simulink model "mrefrobotarm_previous_y_previous_u_previous_ref_cex_2"  (R2018b)
settings: Solver=FixedStepAuto  StartTime=0.0  StopTime=20  RelTol=1e-3  AbsTol=1e-6
undefined symbols (not defined in the file or in its folder): cc, options
libraries: neural x462, simulink x2
(part 8 of 18)

== system mrefrobotarm_previous_y_previous_u_previous_ref_cex_2/cex_m1/Layer 3/Delays 1 ==
  "p{3}" : Inport  PortDimensions=30
      mask Display: e = 0.06;c1 = [120 230 180]/255;c2 = ([120 230 180]+0)/(256+128);c3 = ([120 230 180]+128)/(256+128);patch([0 1 1 0],[0 0 1 1],c1);patch([0 1 1 1-e 1-e 0+e],[0 0 1 1-e 0+e 0+e],c2);patch([0 0 1 1-e 0+e 0+e],[0 1 1 1-e 1-e 0+e],c3);plot([0 1 1 0 0],[0 0 1 1 0]);
  mux : Mux  Inputs=1
      mask Display: e = 0.06;c1 = [120 150 230]/255;c2 = ([120 150 230]+0)/383;c3 = ([120 150 230]+128)/383;patch([0 1 1 0],[0 0 1 1],c1);patch([0 1 1 1-e 1-e 0+e],[0 0 1 1-e 0+e 0+e],c2);patch([0 0 1 1-e 0+e 0+e],[0 1 1 1-e 1-e 0+e],c3);plot([0 1 1 0 0],[0 0 1 1 0]);disp('Mux')
  "pd{3,2}" : Outport
      mask Display: e = 0.06;c1 = [120 230 180]/255;c2 = ([120 230 180]+0)/(256+128);c3 = ([120 230 180]+128)/(256+128);patch([0 1 1 0],[0 0 1 1],c1);patch([0 1 1 1-e 1-e 0+e],[0 0 1 1-e 0+e 0+e],c2);patch([0 0 1 1-e 0+e 0+e],[0 1 1 1-e 1-e 0+e],c3);plot([0 1 1 0 0],[0 0 1 1 0]);
  wires:
  "p{3}"/1 -> mux/1
  mux/1 -> "pd{3,2}"/1

== system mrefrobotarm_previous_y_previous_u_previous_ref_cex_2/cex_m1/Layer 3/LW{3,2} ==
  "ad{3,2}" : Inport  PortDimensions=30
      mask Display: e = 0.06;c1 = [120 230 180]/255;c2 = ([120 230 180]+0)/(256+128);c3 = ([120 230 180]+128)/(256+128);patch([0 1 1 0],[0 0 1 1],c1);patch([0 1 1 1-e 1-e 0+e],[0 0 1 1-e 0+e 0+e],c2);patch([0 0 1 1-e 0+e 0+e],[0 1 1 1-e 1-e 0+e],c3);plot([0 1 1 0 0],[0 0 1 1 0]);
  "IW{3,2}(1,:)'" : Constant  Value=[0.273559337497494947655241048778407275676727294921875;-0.7756545835412576028744524592184461653232574462890625;-0.2367085924296140897471474318081163801252841949462890625;-0.07780558994367196834485156387017923407256603240966796875;0.62547021966759819289194410885102115571498870849609375;-0.042949116212649039725501864950274466536939144134521484375;-0.0115378064817653024076715695400707772932946681976318359375;-0.1916034773301610594220534267151379026472568511962890625;0.07545572263788587197286261698536691255867481231689453125;-0.342221555072600935876181438288767822086811065673828125;0.05574493159312048085052282431206549517810344696044921875;-0.118390555813133235840695078877615742385387420654296875;0.405364924953283967123951470057363621890544891357421875;-0.62424190657044953400856002190266735851764678955078125;0.267676026784579856876433723300579003989696502685546875;-0.53578877848254624627344355758395977318286895751953125;-0.393016319594194307729395632122759707272052764892578125;0.204836160849805881678520336208748631179332733154296875;0.1641507664097359986410396004430367611348628997802734375;0.34723625620254361390237818341120146214962005615234375;0.00875153796303594112837576091123992227949202060699462890625;-0.035480681395222139762335444856944377534091472625732421875;0.021397552117908107127686179183001513592898845672607421875;-0.300775979439210860988396234461106359958648681640625;-0.277260526293208686698932297076680697500705718994140625;-0.09496793333009435900127215290922322310507297515869140625;0.01226152538563072928734509758896820130757987499237060546875;0.051278382491689360189734969708297285251319408416748046875;0.86445975923971551946323188531096093356609344482421875;-0.36925297458121264515540360662271268665790557861328125]
      mask Display: e = 0.06;c1 = [120 150 230]/255;c2 = ([120 150 230]+0)/383;c3 = ([120 150 230]+128)/383;patch([0 1 1 0],[0 0 1 1],c1);patch([0 1 1 1-e 1-e 0+e],[0 0 1 1-e 0+e 0+e],c2);patch([0 0 1 1-e 0+e 0+e],[0 1 1 1-e 1-e 0+e],c3);plot([0 1 1 0 0],[0 0 1 1 0]);disp('weights');
  Mux : Mux  Inputs=1
      mask Display: e = 0.06;c1 = [120 150 230]/255;c2 = ([120 150 230]+0)/383;c3 = ([120 150 230]+128)/383;patch([0 1 1 0],[0 0 1 1],c1);patch([0 1 1 1-e 1-e 0+e],[0 0 1 1-e 0+e 0+e],c2);patch([0 0 1 1-e 0+e 0+e],[0 1 1 1-e 1-e 0+e],c3);plot([0 1 1 0 0],[0 0 1 1 0]);disp('Mux');
  dotprod1 : neural/Weight Functions/dotprod
  "lz{3,2}" : Outport
      mask Display: e = 0.06;c1 = [120 230 180]/255;c2 = ([120 230 180]+0)/(256+128);c3 = ([120 230 180]+128)/(256+128);patch([0 1 1 0],[0 0 1 1],c1);patch([0 1 1 1-e 1-e 0+e],[0 0 1 1-e 0+e 0+e],c2);patch([0 0 1 1-e 0+e 0+e],[0 1 1 1-e 1-e 0+e],c3);plot([0 1 1 0 0],[0 0 1 1 0]);
  wires:
  "IW{3,2}(1,:)'"/1 -> dotprod1/1
  "ad{3,2}"/1 -> dotprod1/2
  dotprod1/1 -> Mux/1
  Mux/1 -> "lz{3,2}"/1

== system mrefrobotarm_previous_y_previous_u_previous_ref_cex_2/cex_m1_old/Layer 1/Delays 1 ==
  "p{1}" : Inport  PortDimensions=10
      mask Display: e = 0.06;c1 = [120 230 180]/255;c2 = ([120 230 180]+0)/(256+128);c3 = ([120 230 180]+128)/(256+128);patch([0 1 1 0],[0 0 1 1],c1);patch([0 1 1 1-e 1-e 0+e],[0 0 1 1-e 0+e 0+e],c2);patch([0 0 1 1-e 0+e 0+e],[0 1 1 1-e 1-e 0+e],c3);plot([0 1 1 0 0],[0 0 1 1 0]);
  mux : Mux  Inputs=1
      mask Display: e = 0.06;c1 = [120 150 230]/255;c2 = ([120 150 230]+0)/383;c3 = ([120 150 230]+128)/383;patch([0 1 1 0],[0 0 1 1],c1);patch([0 1 1 1-e 1-e 0+e],[0 0 1 1-e 0+e 0+e],c2);patch([0 0 1 1-e 0+e 0+e],[0 1 1 1-e 1-e 0+e],c3);plot([0 1 1 0 0],[0 0 1 1 0]);disp('Mux')
  "pd{1,1}" : Outport
      mask Display: e = 0.06;c1 = [120 230 180]/255;c2 = ([120 230 180]+0)/(256+128);c3 = ([120 230 180]+128)/(256+128);patch([0 1 1 0],[0 0 1 1],c1);patch([0 1 1 1-e 1-e 0+e],[0 0 1 1-e 0+e 0+e],c2);patch([0 0 1 1-e 0+e 0+e],[0 1 1 1-e 1-e 0+e],c3);plot([0 1 1 0 0],[0 0 1 1 0]);
  wires:
  "p{1}"/1 -> mux/1
  mux/1 -> "pd{1,1}"/1

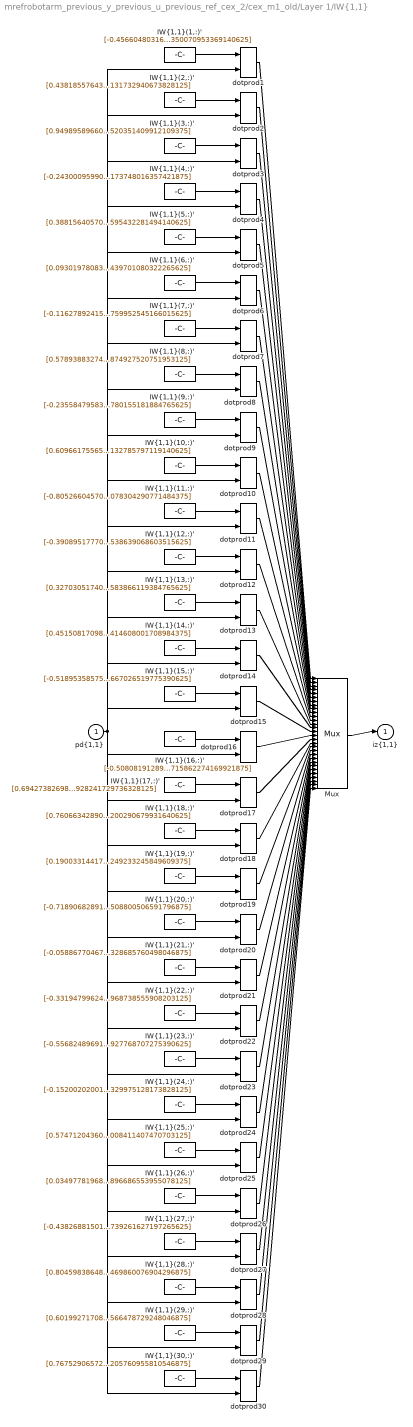
== system mrefrobotarm_previous_y_previous_u_previous_ref_cex_2/cex_m1_old/Layer 1/IW{1,1} ==
  "pd{1,1}" : Inport  PortDimensions=10
      mask Display: e = 0.06;c1 = [120 230 180]/255;c2 = ([120 230 180]+0)/(256+128);c3 = ([120 230 180]+128)/(256+128);patch([0 1 1 0],[0 0 1 1],c1);patch([0 1 1 1-e 1-e 0+e],[0 0 1 1-e 0+e 0+e],c2);patch([0 0 1 1-e 0+e 0+e],[0 1 1 1-e 1-e 0+e],c3);plot([0 1 1 0 0],[0 0 1 1 0]);
  "IW{1,1}(1,:)'" : Constant  Value=[-0.456604803168614292729898807010613381862640380859375;-0.337127164338302864887708665264653973281383514404296875;-0.09380605620231612096215911833496647886931896209716796875;0.4813255060015799724482121746405027806758880615234375;-0.51828644978876658999666915406123735010623931884765625;-0.360214664462510547604523480913485400378704071044921875;-0.1613924539391769774621110400403267703950405120849609375;-0.45837538185699278070472928447998128831386566162109375;0.98037037066747012570289143695845268666744232177734375;0.369741124667328835418089738595881499350070953369140625]
      mask Display: e = 0.06;c1 = [120 150 230]/255;c2 = ([120 150 230]+0)/383;c3 = ([120 150 230]+128)/383;patch([0 1 1 0],[0 0 1 1],c1);patch([0 1 1 1-e 1-e 0+e],[0 0 1 1-e 0+e 0+e],c2);patch([0 0 1 1-e 0+e 0+e],[0 1 1 1-e 1-e 0+e],c3);plot([0 1 1 0 0],[0 0 1 1 0]);disp('Weights');
  "IW{1,1}(10,:)'" : Constant  Value=[0.60966175565233104993723145526018925011157989501953125;-0.78590103009985778914625598190468735992908477783203125;0.67529278324963026847171931876800954341888427734375;-0.538121168742959010700133148930035531520843505859375;0.6927400264329157675291526174987666308879852294921875;0.340750317165999572210921542136929929256439208984375;0.40556995495471770407647227330016903579235076904296875;-0.0484033308948597085219489599694497883319854736328125;-0.164300434052266519646678943900042213499546051025390625;-0.58676709523571946025555234882631339132785797119140625]
      mask Display: e = 0.06;c1 = [120 150 230]/255;c2 = ([120 150 230]+0)/383;c3 = ([120 150 230]+128)/383;patch([0 1 1 0],[0 0 1 1],c1);patch([0 1 1 1-e 1-e 0+e],[0 0 1 1-e 0+e 0+e],c2);patch([0 0 1 1-e 0+e 0+e],[0 1 1 1-e 1-e 0+e],c3);plot([0 1 1 0 0],[0 0 1 1 0]);disp('Weights');
  "IW{1,1}(11,:)'" : Constant  Value=[-0.8052660457061115995003319767420180141925811767578125;-0.390578940383738970609783791587688028812408447265625;-0.307426974497562233157310629394487477838993072509765625;0.18849807820618769138576453769928775727748870849609375;-0.39029554181874825946607643345487304031848907470703125;0.50189857658144487739804162629297934472560882568359375;-1.3944440472362054084243254692410118877887725830078125;0.052818878114326554829016657777174259535968303680419921875;0.52703996195776647848418861030950210988521575927734375;0.64912684710533896659256924976943992078304290771484375]
      mask Display: e = 0.06;c1 = [120 150 230]/255;c2 = ([120 150 230]+0)/383;c3 = ([120 150 230]+128)/383;patch([0 1 1 0],[0 0 1 1],c1);patch([0 1 1 1-e 1-e 0+e],[0 0 1 1-e 0+e 0+e],c2);patch([0 0 1 1-e 0+e 0+e],[0 1 1 1-e 1-e 0+e],c3);plot([0 1 1 0 0],[0 0 1 1 0]);disp('Weights');
  "IW{1,1}(12,:)'" : Constant  Value=[-0.39089517770435111554405693823355250060558319091796875;0.87652548903037030836316034765332005918025970458984375;-0.86066296477683745802522707890602760016918182373046875;0.2435082234393515232540039505693130195140838623046875;-0.01260654893496855090406771893185577937401831150054931640625;0.58088923822424043397205650762771256268024444580078125;0.79790414878794369002434905269183218479156494140625;-0.321088353238704937719916188143542967736721038818359375;0.46829250187147308803758960493723861873149871826171875;0.105276077235084086769489886137307621538639068603515625]
      mask Display: e = 0.06;c1 = [120 150 230]/255;c2 = ([120 150 230]+0)/383;c3 = ([120 150 230]+128)/383;patch([0 1 1 0],[0 0 1 1],c1);patch([0 1 1 1-e 1-e 0+e],[0 0 1 1-e 0+e 0+e],c2);patch([0 0 1 1-e 0+e 0+e],[0 1 1 1-e 1-e 0+e],c3);plot([0 1 1 0 0],[0 0 1 1 0]);disp('Weights');
  "IW{1,1}(13,:)'" : Constant  Value=[0.327030517403528120379263555150828324258327484130859375;-0.85196641992506927376638259374885819852352142333984375;-0.3458136539724006031093495039385743439197540283203125;0.56880574832738928225950303385616280138492584228515625;0.060222487967785363893735706142251729033887386322021484375;0.0444849469077064352262596003129146993160247802734375;-0.6806078651776008570095655159093439579010009765625;0.443959968651114367244048253269284032285213470458984375;-0.23601846855789110346535153439617715775966644287109375;0.60569342459776598364129540641442872583866119384765625]
      mask Display: e = 0.06;c1 = [120 150 230]/255;c2 = ([120 150 230]+0)/383;c3 = ([120 150 230]+128)/383;patch([0 1 1 0],[0 0 1 1],c1);patch([0 1 1 1-e 1-e 0+e],[0 0 1 1-e 0+e 0+e],c2);patch([0 0 1 1-e 0+e 0+e],[0 1 1 1-e 1-e 0+e],c3);plot([0 1 1 0 0],[0 0 1 1 0]);disp('Weights');
  "IW{1,1}(14,:)'" : Constant  Value=[0.4515081709834014578319738575373776257038116455078125;-0.8989078222605810797318781624198891222476959228515625;0.454253767808243280601487867897958494722843170166015625;-0.197872388974969226627109719629515893757343292236328125;-0.284539642220156763219307549661607481539249420166015625;0.8759306435735558782340604011551477015018463134765625;-0.1785360111457083842623205782729201018810272216796875;-0.2001588807255618995828427841843222267925739288330078125;0.53520676898232066864835587693960405886173248291015625;0.94559736423401774541019904063432477414608001708984375]
      mask Display: e = 0.06;c1 = [120 150 230]/255;c2 = ([120 150 230]+0)/383;c3 = ([120 150 230]+128)/383;patch([0 1 1 0],[0 0 1 1],c1);patch([0 1 1 1-e 1-e 0+e],[0 0 1 1-e 0+e 0+e],c2);patch([0 0 1 1-e 0+e 0+e],[0 1 1 1-e 1-e 0+e],c3);plot([0 1 1 0 0],[0 0 1 1 0]);disp('Weights');
  "IW{1,1}(15,:)'" : Constant  Value=[-0.518953585756852131538607864058576524257659912109375;-0.8287693770535684567590806182124651968479156494140625;0.61069653280025570918354560490115545690059661865234375;0.455111773439323352707930325777851976454257965087890625;0.61500607296115672451009004362276755273342132568359375;-0.36577833850321705977393094144645147025585174560546875;0.1471285663392648823677433256307267583906650543212890625;-0.5784088886907132742720705209649167954921722412109375;0.07806634820889439552171751302012125961482524871826171875;0.69003575602860645066272127223783172667026519775390625]
      mask Display: e = 0.06;c1 = [120 150 230]/255;c2 = ([120 150 230]+0)/383;c3 = ([120 150 230]+128)/383;patch([0 1 1 0],[0 0 1 1],c1);patch([0 1 1 1-e 1-e 0+e],[0 0 1 1-e 0+e 0+e],c2);patch([0 0 1 1-e 0+e 0+e],[0 1 1 1-e 1-e 0+e],c3);plot([0 1 1 0 0],[0 0 1 1 0]);disp('Weights');
  "IW{1,1}(16,:)'" : Constant  Value=[-0.5080819128972311471414968764293007552623748779296875;0.064120829622686448256985158877796493470668792724609375;-0.1899203040905295403195651715577696450054645538330078125;0.028825660348881392003317358785352553240954875946044921875;0.8950447302793678172605496001779101788997650146484375;-0.6350696078018034373968703221180476248264312744140625;0.69836883039490371682944669373682700097560882568359375;-0.2994246938013576109227642518817447125911712646484375;0.56725449704477826085025071733980439603328704833984375;-0.37050563293872595949096648837439715862274169921875]
      mask Display: e = 0.06;c1 = [120 150 230]/255;c2 = ([120 150 230]+0)/383;c3 = ([120 150 230]+128)/383;patch([0 1 1 0],[0 0 1 1],c1);patch([0 1 1 1-e 1-e 0+e],[0 0 1 1-e 0+e 0+e],c2);patch([0 0 1 1-e 0+e 0+e],[0 1 1 1-e 1-e 0+e],c3);plot([0 1 1 0 0],[0 0 1 1 0]);disp('Weights');
  "IW{1,1}(17,:)'" : Constant  Value=[0.69427382698219963774732832462177611887454986572265625;-0.488497940847307077216754578330437652766704559326171875;0.76921833962025198960787975011044181883335113525390625;-0.91091754430127747088619116766494698822498321533203125;-0.1745040246724469945593938291494851000607013702392578125;0.0066101774826527737172199294946040026843547821044921875;0.453900939435363082186114525029552169144153594970703125;0.07387565171452577239552539367650751955807209014892578125;0.69920054733834613447385208928608335554599761962890625;-0.1244791951685582376274652460779179818928241729736328125]
      mask Display: e = 0.06;c1 = [120 150 230]/255;c2 = ([120 150 230]+0)/383;c3 = ([120 150 230]+128)/383;patch([0 1 1 0],[0 0 1 1],c1);patch([0 1 1 1-e 1-e 0+e],[0 0 1 1-e 0+e 0+e],c2);patch([0 0 1 1-e 0+e 0+e],[0 1 1 1-e 1-e 0+e],c3);plot([0 1 1 0 0],[0 0 1 1 0]);disp('Weights');
  "IW{1,1}(18,:)'" : Constant  Value=[0.76066342890209115434885234208195470273494720458984375;0.51801825655466082753974887964432127773761749267578125;0.91420683388085322018667966403882019221782684326171875;-0.49680504344115739012721633116598241031169891357421875;0.926993167798115802469283153186552226543426513671875;0.38135095924055273375330443741404451429843902587890625;0.774530566058326375156184440129436552524566650390625;-0.533047430909843189539287777733989059925079345703125;-0.0174997496667618490651108231759280897676944732666015625;0.355609156460071462735328395865508355200290679931640625]
      mask Display: e = 0.06;c1 = [120 150 230]/255;c2 = ([120 150 230]+0)/383;c3 = ([120 150 230]+128)/383;patch([0 1 1 0],[0 0 1 1],c1);patch([0 1 1 1-e 1-e 0+e],[0 0 1 1-e 0+e 0+e],c2);patch([0 0 1 1-e 0+e 0+e],[0 1 1 1-e 1-e 0+e],c3);plot([0 1 1 0 0],[0 0 1 1 0]);disp('Weights');
  "IW{1,1}(19,:)'" : Constant  Value=[0.1900331441796630771445819618747918866574764251708984375;0.53025746047892752255137338579515926539897918701171875;-0.395669897903047240728113820296130143105983734130859375;-0.6907448236475797198608006510767154395580291748046875;0.36487531515756810307493651635013520717620849609375;-0.84679918588567992809856832536752335727214813232421875;0.292288624186119172509989994068746455013751983642578125;0.1586375850129098097340829554013907909393310546875;0.041807865616759622151565878311885171569883823394775390625;0.95747807301410892133475272203213535249233245849609375]
      mask Display: e = 0.06;c1 = [120 150 230]/255;c2 = ([120 150 230]+0)/383;c3 = ([120 150 230]+128)/383;patch([0 1 1 0],[0 0 1 1],c1);patch([0 1 1 1-e 1-e 0+e],[0 0 1 1-e 0+e 0+e],c2);patch([0 0 1 1-e 0+e 0+e],[0 1 1 1-e 1-e 0+e],c3);plot([0 1 1 0 0],[0 0 1 1 0]);disp('Weights');
  "IW{1,1}(2,:)'" : Constant  Value=[0.438185576430030920835889673981000669300556182861328125;0.63169008794116454641454083684948273003101348876953125;-0.690212126796364344727408024482429027557373046875;0.126418981169538924280715264103491790592670440673828125;-0.78081879756354766186632332392036914825439453125;0.036441711512395225103233542540692724287509918212890625;0.80831443252255363862701642574393190443515777587890625;-0.5695381261843135423106332382303662598133087158203125;0.372937259042779134521339301500120200216770172119140625;0.76200855637333220204965300581534393131732940673828125]
      mask Display: e = 0.06;c1 = [120 150 230]/255;c2 = ([120 150 230]+0)/383;c3 = ([120 150 230]+128)/383;patch([0 1 1 0],[0 0 1 1],c1);patch([0 1 1 1-e 1-e 0+e],[0 0 1 1-e 0+e 0+e],c2);patch([0 0 1 1-e 0+e 0+e],[0 1 1 1-e 1-e 0+e],c3);plot([0 1 1 0 0],[0 0 1 1 0]);disp('Weights');
  "IW{1,1}(20,:)'" : Constant  Value=[-0.71890682891750745664438682069885544478893280029296875;0.323748238412146893683285497900214977562427520751953125;-0.4350383245811233479116708622314035892486572265625;-0.098115153846664859838000438685412518680095672607421875;0.332374149245302785704581083336961455643177032470703125;0.665347500692802018562588273198343813419342041015625;-0.996297270814632707214286710950545966625213623046875;0.22478310077883134621146155041060410439968109130859375;0.07675674847099771269665069439724902622401714324951171875;-0.39635430828158735305777327084797434508800506591796875]
      mask Display: e = 0.06;c1 = [120 150 230]/255;c2 = ([120 150 230]+0)/383;c3 = ([120 150 230]+128)/383;patch([0 1 1 0],[0 0 1 1],c1);patch([0 1 1 1-e 1-e 0+e],[0 0 1 1-e 0+e 0+e],c2);patch([0 0 1 1-e 0+e 0+e],[0 1 1 1-e 1-e 0+e],c3);plot([0 1 1 0 0],[0 0 1 1 0]);disp('Weights');
  "IW{1,1}(21,:)'" : Constant  Value=[-0.058867704679459571803779027732161921449005603790283203125;0.318806140277555438711232227433356456458568572998046875;0.5514498503440876664427605646778829395771026611328125;-0.843025654861124795758087202557362616062164306640625;0.42766102343846423838868986422312445938587188720703125;-0.73504404909710008286793936349567957222461700439453125;-0.76913120987454008936623495173989795148372650146484375;0.0070151290944123097237383746005434659309685230255126953125;0.79142247809240073852521391017944552004337310791015625;0.283648015671342956789402478534611873328685760498046875]
      mask Display: e = 0.06;c1 = [120 150 230]/255;c2 = ([120 150 230]+0)/383;c3 = ([120 150 230]+128)/383;patch([0 1 1 0],[0 0 1 1],c1);patch([0 1 1 1-e 1-e 0+e],[0 0 1 1-e 0+e 0+e],c2);patch([0 0 1 1-e 0+e 0+e],[0 1 1 1-e 1-e 0+e],c3);plot([0 1 1 0 0],[0 0 1 1 0]);disp('Weights');
  "IW{1,1}(22,:)'" : Constant  Value=[-0.331947996244390031161941578830010257661342620849609375;-0.2268747378868123387718469530227594077587127685546875;0.61424614718336278951227313882554881274700164794921875;-0.57641523587598830768996549522853456437587738037109375;-0.6983402399747113964423306242679245769977569580078125;0.73226198126729824533498458549729548394680023193359375;0.6098680765245083623682376128272153437137603759765625;-0.81514112188509824097337741477531380951404571533203125;0.5435968206353025689026026157080195844173431396484375;0.383290174564916708010997581368428654968738555908203125]
      mask Display: e = 0.06;c1 = [120 150 230]/255;c2 = ([120 150 230]+0)/383;c3 = ([120 150 230]+128)/383;patch([0 1 1 0],[0 0 1 1],c1);patch([0 1 1 1-e 1-e 0+e],[0 0 1 1-e 0+e 0+e],c2);patch([0 0 1 1-e 0+e 0+e],[0 1 1 1-e 1-e 0+e],c3);plot([0 1 1 0 0],[0 0 1 1 0]);disp('Weights');
  "IW{1,1}(23,:)'" : Constant  Value=[-0.55682489691597714109860817188746295869350433349609375;0.3971753371402726440209107749979011714458465576171875;-0.94266284346768802748783855349756777286529541015625;0.2233454508858634113277474853020976297557353973388671875;-0.78108602978100460934030024873209185898303985595703125;-0.355621419148077710925548444720334373414516448974609375;1.04371286491103543170311240828596055507659912109375;-0.575221360774758050382615692797116935253143310546875;-0.040419337166701672925395172342177829705178737640380859375;0.60627576039757935522089837832027114927768707275390625]
      mask Display: e = 0.06;c1 = [120 150 230]/255;c2 = ([120 150 230]+0)/383;c3 = ([120 150 230]+128)/383;patch([0 1 1 0],[0 0 1 1],c1);patch([0 1 1 1-e 1-e 0+e],[0 0 1 1-e 0+e 0+e],c2);patch([0 0 1 1-e 0+e 0+e],[0 1 1 1-e 1-e 0+e],c3);plot([0 1 1 0 0],[0 0 1 1 0]);disp('Weights');
  "IW{1,1}(24,:)'" : Constant  Value=[-0.152002020012920124880650973864248953759670257568359375;0.267355262853008091017414926682249642908573150634765625;0.3681014583243105153798069295589812099933624267578125;0.60380396349835752101142816172796301543712615966796875;-0.2240663683106254300270165913389064371585845947265625;-0.2118074012804891104178039995531435124576091766357421875;0.61766038108176901655355095499544404447078704833984375;-0.10347664558279710822485952803617692552506923675537109375;1.0088377721471577519452011983958072960376739501953125;-0.296533638802529697642285100300796329975128173828125]
      mask Display: e = 0.06;c1 = [120 150 230]/255;c2 = ([120 150 230]+0)/383;c3 = ([120 150 230]+128)/383;patch([0 1 1 0],[0 0 1 1],c1);patch([0 1 1 1-e 1-e 0+e],[0 0 1 1-e 0+e 0+e],c2);patch([0 0 1 1-e 0+e 0+e],[0 1 1 1-e 1-e 0+e],c3);plot([0 1 1 0 0],[0 0 1 1 0]);disp('Weights');
  "IW{1,1}(25,:)'" : Constant  Value=[0.5747120436081643024550658083171583712100982666015625;-1.0586365897313012585101432705414481461048126220703125;0.09387458902065796972902234074354055337607860565185546875;-0.052016654662084292615187308683744049631059169769287109375;-0.4780536664053312012612195758265443146228790283203125;0.9806526512700610709316606516949832439422607421875;-0.1030533823984588204236700903493328951299190521240234375;-0.16531964088011064095695701325894333422183990478515625;0.32575705366995766354420993593521416187286376953125;-0.8915608655361009216022694090497680008411407470703125]
      mask Display: e = 0.06;c1 = [120 150 230]/255;c2 = ([120 150 230]+0)/383;c3 = ([120 150 230]+128)/383;patch([0 1 1 0],[0 0 1 1],c1);patch([0 1 1 1-e 1-e 0+e],[0 0 1 1-e 0+e 0+e],c2);patch([0 0 1 1-e 0+e 0+e],[0 1 1 1-e 1-e 0+e],c3);plot([0 1 1 0 0],[0 0 1 1 0]);disp('Weights');
  "IW{1,1}(26,:)'" : Constant  Value=[0.0349778196856112277846051483720657415688037872314453125;1.0546893984497180962733864362235181033611297607421875;0.5113372359302978953365936831687577068805694580078125;-0.20958359966499229276593041504384018480777740478515625;-0.45906996765058216691812731369282118976116180419921875;-0.350427826420348365044077354468754492700099945068359375;0.91643043413432445642996526657952927052974700927734375;-0.6214855448244855917749873697175644338130950927734375;-0.52581356029745618396731288157752715051174163818359375;-0.06278736980947492718474478579082642681896686553955078125]
      mask Display: e = 0.06;c1 = [120 150 230]/255;c2 = ([120 150 230]+0)/383;c3 = ([120 150 230]+128)/383;patch([0 1 1 0],[0 0 1 1],c1);patch([0 1 1 1-e 1-e 0+e],[0 0 1 1-e 0+e 0+e],c2);patch([0 0 1 1-e 0+e 0+e],[0 1 1 1-e 1-e 0+e],c3);plot([0 1 1 0 0],[0 0 1 1 0]);disp('Weights');
  "IW{1,1}(27,:)'" : Constant  Value=[-0.43826881501622050318900392085197381675243377685546875;-0.56314499853929256278917137024109251797199249267578125;0.95485425315337213447719477699138224124908447265625;-0.5166485659506478977931465124129317700862884521484375;-0.40061838248913350657431919898954220116138458251953125;0.479935634958266577054786239386885426938533782958984375;-0.1618372276251738295371751519269309937953948974609375;-0.05277579066387456940834255192385171540081501007080078125;-0.62106660802614099825547100408584810793399810791015625;0.440122852015918886170453561135218478739261627197265625]
      mask Display: e = 0.06;c1 = [120 150 230]/255;c2 = ([120 150 230]+0)/383;c3 = ([120 150 230]+128)/383;patch([0 1 1 0],[0 0 1 1],c1);patch([0 1 1 1-e 1-e 0+e],[0 0 1 1-e 0+e 0+e],c2);patch([0 0 1 1-e 0+e 0+e],[0 1 1 1-e 1-e 0+e],c3);plot([0 1 1 0 0],[0 0 1 1 0]);disp('Weights');
  "IW{1,1}(28,:)'" : Constant  Value=[0.80459838648452908227426405574078671634197235107421875;-0.39597574624890530259335719165392220020294189453125;0.5051526717635905772141313718748278915882110595703125;0.462764824426304677285060051872278563678264617919921875;-1.0628527927973758782087543295347131788730621337890625;1.0194158469405987244016387194278649985790252685546875;0.1563891107817585168771046255642431788146495819091796875;-0.34074100067766710520089645797270350158214569091796875;0.11877365410078043195252206487566581927239894866943359375;0.6321743285716425742037927193450741469860076904296875]
      mask Display: e = 0.06;c1 = [120 150 230]/255;c2 = ([120 150 230]+0)/383;c3 = ([120 150 230]+128)/383;patch([0 1 1 0],[0 0 1 1],c1);patch([0 1 1 1-e 1-e 0+e],[0 0 1 1-e 0+e 0+e],c2);patch([0 0 1 1-e 0+e 0+e],[0 1 1 1-e 1-e 0+e],c3);plot([0 1 1 0 0],[0 0 1 1 0]);disp('Weights');
  "IW{1,1}(29,:)'" : Constant  Value=[0.6019927170858758724847348275943659245967864990234375;0.69170657244695821219693243619985878467559814453125;0.499034749348658601686423708088113926351070404052734375;-1.0176618493873126336524137514061294496059417724609375;0.60101291461199080057298260726383887231349945068359375;-0.51835427775524067772749958749045617878437042236328125;0.8044439507675471556780166793032549321651458740234375;-0.006068804685317574949821040064534827251918613910675048828125;0.29431222403439794010893137965467758476734161376953125;-0.369737442034338836815976492289337329566478729248046875]
      mask Display: e = 0.06;c1 = [120 150 230]/255;c2 = ([120 150 230]+0)/383;c3 = ([120 150 230]+128)/383;patch([0 1 1 0],[0 0 1 1],c1);patch([0 1 1 1-e 1-e 0+e],[0 0 1 1-e 0+e 0+e],c2);patch([0 0 1 1-e 0+e 0+e],[0 1 1 1-e 1-e 0+e],c3);plot([0 1 1 0 0],[0 0 1 1 0]);disp('Weights');
  "IW{1,1}(3,:)'" : Constant  Value=[0.94989589660867890241746636093012057244777679443359375;-0.57924800832076517309587870840914547443389892578125;-0.046607459863546842060433306187405833043158054351806640625;-0.79051877700239303603524376740097068250179290771484375;-0.64125965673198981331637469338602386415004730224609375;0.2309291635995582570028972213549423031508922576904296875;0.2109310150735631272933545687919831834733486175537109375;0.77163485474802950836448189875227399170398712158203125;0.568772548565844804357993780286051332950592041015625;0.45832118390900367099760615019476972520351409912109375]
      mask Display: e = 0.06;c1 = [120 150 230]/255;c2 = ([120 150 230]+0)/383;c3 = ([120 150 230]+128)/383;patch([0 1 1 0],[0 0 1 1],c1);patch([0 1 1 1-e 1-e 0+e],[0 0 1 1-e 0+e 0+e],c2);patch([0 0 1 1-e 0+e 0+e],[0 1 1 1-e 1-e 0+e],c3);plot([0 1 1 0 0],[0 0 1 1 0]);disp('Weights');
  "IW{1,1}(30,:)'" : Constant  Value=[0.7675290657211746303545396585832349956035614013671875;-0.60977897745089182368616320673027075827121734619140625;0.3177646953856301248464433228946290910243988037109375;-0.218306511252900070640947660649544559419155120849609375;-0.848280309521165509778484192793257534503936767578125;0.644065013886538029197481591836549341678619384765625;0.47014779111612625683846999891102313995361328125;0.090820289685668298407250631498754955828189849853515625;-0.483763960227027778326913676210097037255764007568359375;0.69749234259775316768781294740620069205760955810546875]
      mask Display: e = 0.06;c1 = [120 150 230]/255;c2 = ([120 150 230]+0)/383;c3 = ([120 150 230]+128)/383;patch([0 1 1 0],[0 0 1 1],c1);patch([0 1 1 1-e 1-e 0+e],[0 0 1 1-e 0+e 0+e],c2);patch([0 0 1 1-e 0+e 0+e],[0 1 1 1-e 1-e 0+e],c3);plot([0 1 1 0 0],[0 0 1 1 0]);disp('Weights');
  "IW{1,1}(4,:)'" : Constant  Value=[-0.243000959900743496167052626333315856754779815673828125;0.699502893171616069167839668807573616504669189453125;0.1076127188643337950768597011119709350168704986572265625;-0.803046733517962518789090609061531722545623779296875;-0.307357091252833447558856505565927363932132720947265625;0.7864449563716691127268632044433616101741790771484375;-0.5759099168746109054239923352724872529506683349609375;0.229400645563350547018188763104262761771678924560546875;-0.1921506876559379295432705703206011094152927398681640625;0.7260042265290926888354761103983037173748016357421875]
      mask Display: e = 0.06;c1 = [120 150 230]/255;c2 = ([120 150 230]+0)/383;c3 = ([120 150 230]+128)/383;patch([0 1 1 0],[0 0 1 1],c1);patch([0 1 1 1-e 1-e 0+e],[0 0 1 1-e 0+e 0+e],c2);patch([0 0 1 1-e 0+e 0+e],[0 1 1 1-e 1-e 0+e],c3);plot([0 1 1 0 0],[0 0 1 1 0]);disp('Weights');
  "IW{1,1}(5,:)'" : Constant  Value=[0.388156405700810502867881268684868700802326202392578125;0.2257297732933698508617226252681575715541839599609375;-0.67674396680373671841834948281757533550262451171875;-0.2805211140532291036464584976783953607082366943359375;-0.191229707050033892468121621277532540261745452880859375;0.7051082587260892875491435916046611964702606201171875;0.262178825133071502495596405424294061958789825439453125;0.2457852725429826301617453054859652183949947357177734375;0.83548352838854300639326311284094117581844329833984375;0.6996973285824383825826089378097094595432281494140625]
      mask Display: e = 0.06;c1 = [120 150 230]/255;c2 = ([120 150 230]+0)/383;c3 = ([120 150 230]+128)/383;patch([0 1 1 0],[0 0 1 1],c1);patch([0 1 1 1-e 1-e 0+e],[0 0 1 1-e 0+e 0+e],c2);patch([0 0 1 1-e 0+e 0+e],[0 1 1 1-e 1-e 0+e],c3);plot([0 1 1 0 0],[0 0 1 1 0]);disp('Weights');
  "IW{1,1}(6,:)'" : Constant  Value=[0.09301978083392596630130100265887449495494365692138671875;0.9726701091526799292097393845324404537677764892578125;-0.61223252158373775433375385546241886913776397705078125;0.2493732790085052275497190521491575054824352264404296875;0.51580802367886546822006721413345076143741607666015625;-0.143754413302846939526347114224336110055446624755859375;0.062331035450019618704420309995839488692581653594970703125;0.80125918071851154333984368349774740636348724365234375;0.5689011672031731858822922731633298099040985107421875;-0.7747518594622369025870511904940940439701080322265625]
      mask Display: e = 0.06;c1 = [120 150 230]/255;c2 = ([120 150 230]+0)/383;c3 = ([120 150 230]+128)/383;patch([0 1 1 0],[0 0 1 1],c1);patch([0 1 1 1-e 1-e 0+e],[0 0 1 1-e 0+e 0+e],c2);patch([0 0 1 1-e 0+e 0+e],[0 1 1 1-e 1-e 0+e],c3);plot([0 1 1 0 0],[0 0 1 1 0]);disp('Weights');
  "IW{1,1}(7,:)'" : Constant  Value=[-0.116278924154781193589514032282750122249126434326171875;-0.558107690910552012297785040573216974735260009765625;0.306770330448174533000127439663629047572612762451171875;0.481439420237415038883455054019577801227569580078125;-0.62273588170325389068437971218372695147991180419921875;-0.0210564363500323446787287906545316218398511409759521484375;0.806668981632385762026160591631196439266204833984375;-0.08530034802376697256054427498384029604494571685791015625;-1.04329976505287191912429989315569400787353515625;0.349826242822306510138474777704686857759952545166015625]
      mask Display: e = 0.06;c1 = [120 150 230]/255;c2 = ([120 150 230]+0)/383;c3 = ([120 150 230]+128)/383;patch([0 1 1 0],[0 0 1 1],c1);patch([0 1 1 1-e 1-e 0+e],[0 0 1 1-e 0+e 0+e],c2);patch([0 0 1 1-e 0+e 0+e],[0 1 1 1-e 1-e 0+e],c3);plot([0 1 1 0 0],[0 0 1 1 0]);disp('Weights');
  "IW{1,1}(8,:)'" : Constant  Value=[0.57893883274759938561970784576260484755039215087890625;-0.631794753968332400972940376959741115570068359375;0.61377448556544778046628607626189477741718292236328125;-0.24743734310279263954868156361044384539127349853515625;0.685481692558628008526966368663124740123748779296875;-0.5562688244819822269704445716342888772487640380859375;-0.58281545571056503352025401909486390650272369384765625;0.872436655985315834271887069917283952236175537109375;-0.727531025695643318584870939957909286022186279296875;-0.14352958591145725808502220388618297874927520751953125]
      mask Display: e = 0.06;c1 = [120 150 230]/255;c2 = ([120 150 230]+0)/383;c3 = ([120 150 230]+128)/383;patch([0 1 1 0],[0 0 1 1],c1);patch([0 1 1 1-e 1-e 0+e],[0 0 1 1-e 0+e 0+e],c2);patch([0 0 1 1-e 0+e 0+e],[0 1 1 1-e 1-e 0+e],c3);plot([0 1 1 0 0],[0 0 1 1 0]);disp('Weights');
  "IW{1,1}(9,:)'" : Constant  Value=[-0.2355847958392153496109955312931560911238193511962890625;0.2775337753692295184038130173576064407825469970703125;0.79443059838741436617937097253161482512950897216796875;-0.7332221181677780474927885734359733760356903076171875;1.09127230197237690134670629049651324748992919921875;-0.80075294497843574337281324915238656103610992431640625;-0.3440831422867225430906046312884427607059478759765625;0.6179798556164992628936261098715476691722869873046875;-0.348884416455360002462526836097822524607181549072265625;-0.08794648399861272614064233721364871598780155181884765625]
      mask Display: e = 0.06;c1 = [120 150 230]/255;c2 = ([120 150 230]+0)/383;c3 = ([120 150 230]+128)/383;patch([0 1 1 0],[0 0 1 1],c1);patch([0 1 1 1-e 1-e 0+e],[0 0 1 1-e 0+e 0+e],c2);patch([0 0 1 1-e 0+e 0+e],[0 1 1 1-e 1-e 0+e],c3);plot([0 1 1 0 0],[0 0 1 1 0]);disp('Weights');
  Mux : Mux  Inputs=30
      mask Display: e = 0.06;c1 = [120 150 230]/255;c2 = ([120 150 230]+0)/383;c3 = ([120 150 230]+128)/383;patch([0 1 1 0],[0 0 1 1],c1);patch([0 1 1 1-e 1-e 0+e],[0 0 1 1-e 0+e 0+e],c2);patch([0 0 1 1-e 0+e 0+e],[0 1 1 1-e 1-e 0+e],c3);plot([0 1 1 0 0],[0 0 1 1 0]);disp('Mux');
  dotprod{1..30} (30 alike) : neural/Weight Functions/dotprod
  "iz{1,1}" : Outport
      mask Display: e = 0.06;c1 = [120 230 180]/255;c2 = ([120 230 180]+0)/(256+128);c3 = ([120 230 180]+128)/(256+128);patch([0 1 1 0],[0 0 1 1],c1);patch([0 1 1 1-e 1-e 0+e],[0 0 1 1-e 0+e 0+e],c2);patch([0 0 1 1-e 0+e 0+e],[0 1 1 1-e 1-e 0+e],c3);plot([0 1 1 0 0],[0 0 1 1 0]);
  wires:
  "IW{1,1}(1,:)'"/1 -> dotprod1/1
  "pd{1,1}"/1 -> dotprod1/2, dotprod2/2, dotprod3/2, dotprod4/2, dotprod5/2, dotprod6/2, dotprod7/2, dotprod8/2, dotprod9/2, dotprod10/2, dotprod11/2, dotprod12/2, dotprod13/2, dotprod14/2, dotprod15/2, dotprod16/2, dotprod17/2, dotprod18/2, dotprod19/2, dotprod20/2, dotprod21/2, dotprod22/2, dotprod23/2, dotprod24/2, dotprod25/2, dotprod26/2, dotprod27/2, dotprod28/2, dotprod29/2, dotprod30/2
  dotprod1/1 -> Mux/1
  "IW{1,1}(2,:)'"/1 -> dotprod2/1
  dotprod2/1 -> Mux/2
  "IW{1,1}(3,:)'"/1 -> dotprod3/1
  dotprod3/1 -> Mux/3
  "IW{1,1}(4,:)'"/1 -> dotprod4/1
  dotprod4/1 -> Mux/4
  "IW{1,1}(5,:)'"/1 -> dotprod5/1
  dotprod5/1 -> Mux/5
  "IW{1,1}(6,:)'"/1 -> dotprod6/1
  dotprod6/1 -> Mux/6
  "IW{1,1}(7,:)'"/1 -> dotprod7/1
  dotprod7/1 -> Mux/7
  "IW{1,1}(8,:)'"/1 -> dotprod8/1
  dotprod8/1 -> Mux/8
  "IW{1,1}(9,:)'"/1 -> dotprod9/1
  dotprod9/1 -> Mux/9
  "IW{1,1}(10,:)'"/1 -> dotprod10/1
  dotprod10/1 -> Mux/10
  "IW{1,1}(11,:)'"/1 -> dotprod11/1
  dotprod11/1 -> Mux/11
  "IW{1,1}(12,:)'"/1 -> dotprod12/1
  dotprod12/1 -> Mux/12
  "IW{1,1}(13,:)'"/1 -> dotprod13/1
  dotprod13/1 -> Mux/13
  "IW{1,1}(14,:)'"/1 -> dotprod14/1
  dotprod14/1 -> Mux/14
  "IW{1,1}(15,:)'"/1 -> dotprod15/1
  dotprod15/1 -> Mux/15
  "IW{1,1}(16,:)'"/1 -> dotprod16/1
  dotprod16/1 -> Mux/16
  "IW{1,1}(17,:)'"/1 -> dotprod17/1
  dotprod17/1 -> Mux/17
  "IW{1,1}(18,:)'"/1 -> dotprod18/1
  dotprod18/1 -> Mux/18
  "IW{1,1}(19,:)'"/1 -> dotprod19/1
  dotprod19/1 -> Mux/19
  "IW{1,1}(20,:)'"/1 -> dotprod20/1
  dotprod20/1 -> Mux/20
  "IW{1,1}(21,:)'"/1 -> dotprod21/1
  dotprod21/1 -> Mux/21
  "IW{1,1}(22,:)'"/1 -> dotprod22/1
  dotprod22/1 -> Mux/22
  "IW{1,1}(23,:)'"/1 -> dotprod23/1
  dotprod23/1 -> Mux/23
  "IW{1,1}(24,:)'"/1 -> dotprod24/1
  dotprod24/1 -> Mux/24
  "IW{1,1}(25,:)'"/1 -> dotprod25/1
  dotprod25/1 -> Mux/25
  "IW{1,1}(26,:)'"/1 -> dotprod26/1
  dotprod26/1 -> Mux/26
  "IW{1,1}(27,:)'"/1 -> dotprod27/1
  dotprod27/1 -> Mux/27
  "IW{1,1}(28,:)'"/1 -> dotprod28/1
  dotprod28/1 -> Mux/28
  "IW{1,1}(29,:)'"/1 -> dotprod29/1
  dotprod29/1 -> Mux/29
  "IW{1,1}(30,:)'"/1 -> dotprod30/1
  dotprod30/1 -> Mux/30
  Mux/1 -> "iz{1,1}"/1

== system mrefrobotarm_previous_y_previous_u_previous_ref_cex_2/cex_m1_old/Layer 2/Delays 1 ==
  "p{2}" : Inport  PortDimensions=30
      mask Display: e = 0.06;c1 = [120 230 180]/255;c2 = ([120 230 180]+0)/(256+128);c3 = ([120 230 180]+128)/(256+128);patch([0 1 1 0],[0 0 1 1],c1);patch([0 1 1 1-e 1-e 0+e],[0 0 1 1-e 0+e 0+e],c2);patch([0 0 1 1-e 0+e 0+e],[0 1 1 1-e 1-e 0+e],c3);plot([0 1 1 0 0],[0 0 1 1 0]);
  mux : Mux  Inputs=1
      mask Display: e = 0.06;c1 = [120 150 230]/255;c2 = ([120 150 230]+0)/383;c3 = ([120 150 230]+128)/383;patch([0 1 1 0],[0 0 1 1],c1);patch([0 1 1 1-e 1-e 0+e],[0 0 1 1-e 0+e 0+e],c2);patch([0 0 1 1-e 0+e 0+e],[0 1 1 1-e 1-e 0+e],c3);plot([0 1 1 0 0],[0 0 1 1 0]);disp('Mux')
  "pd{2,1}" : Outport
      mask Display: e = 0.06;c1 = [120 230 180]/255;c2 = ([120 230 180]+0)/(256+128);c3 = ([120 230 180]+128)/(256+128);patch([0 1 1 0],[0 0 1 1],c1);patch([0 1 1 1-e 1-e 0+e],[0 0 1 1-e 0+e 0+e],c2);patch([0 0 1 1-e 0+e 0+e],[0 1 1 1-e 1-e 0+e],c3);plot([0 1 1 0 0],[0 0 1 1 0]);
  wires:
  "p{2}"/1 -> mux/1
  mux/1 -> "pd{2,1}"/1
